simulink model "CDMA2000sint_C_etapa4"  (R2012b)
settings: Solver=ode45  StartTime=0.0  StopTime=200  RelTol=1e-3
libraries: commcnvintrlv2 x2, commcnvcod2 x2, commrandsrc2 x1, commsink2 x1
settings Model: Creator=Oti  LastModifiedBy=student
settings DataIOCC: SignalLoggingSaveFormat=ModelDataLogs
settings DebuggingCC: FcnCallInpInsideContextMsg=UseLocalSettings
settings GRTTargetCC: CombineOutputUpdateFcns=off  GRTInterface=on

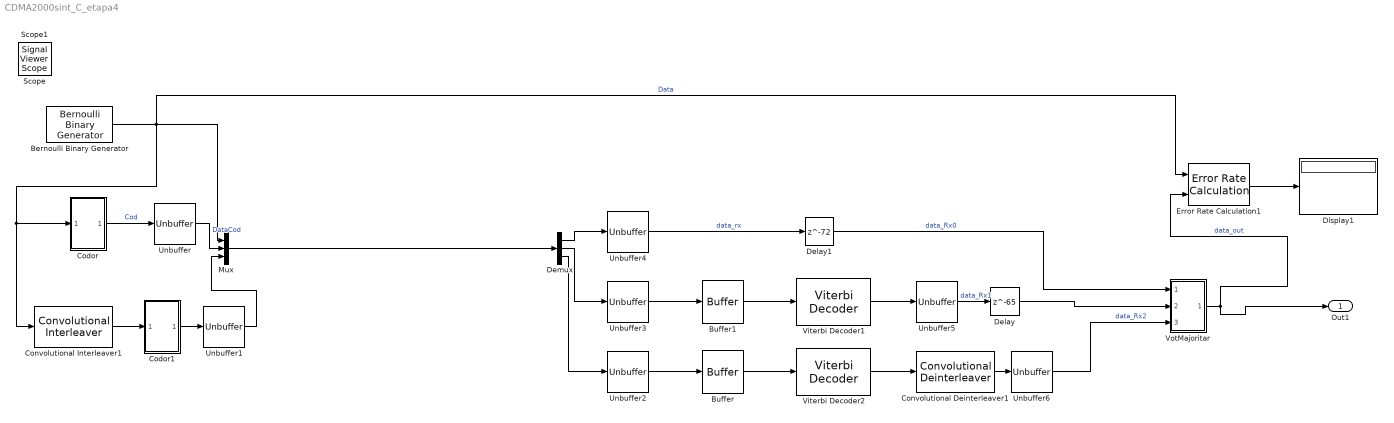
== system CDMA2000sint_C_etapa4 ==
  Bernoulli Binary Generator : commrandsrc2/Bernoulli Binary Generator  P=0.5  seed=61  Ts=1  frameBased=off  sampPerFrame=1  orient=off  outDataType=boolean
  Buffer : Buffer  N=3  TreatMby1Signals=One channel
  Buffer1 : Buffer  N=3  TreatMby1Signals=One channel
  Codor : Subsystem
  Codor1 : Subsystem
  Convolutional Deinterleaver1 : commcnvintrlv2/Convolutional Deinterleaver  N=6  B=2  ic=0
  Convolutional Interleaver1 : commcnvintrlv2/Convolutional Interleaver  N=6  B=2  ic=0
  Delay : Delay  DelayLength=65  SampleTime=1
  Delay1 : Delay  DelayLength=72  SampleTime=1
  Demux : Demux  Outputs=3
  Display1 : Display
  Error Rate Calculation1 : commsink2/Error Rate Calculation  N=72  st_delay=0  cp_mode=Entire frame  subframe=[]  PMode=Port  WsName=ErrorVec  RsMode2=off  stop=off  numErr=100  maxBits=1e6
  Mux : Mux  Inputs=3
  Unbuffer{,1..6} (7 alike) : Unbuffer  SampleBasedProcessing=Same as frame based
  Viterbi Decoder1 : commcnvcod2/Viterbi Decoder  trellis=poly2trellis(4, [13 15 17], 13)  isPunctured=off  punctureVector=[1; 1; 0; 1; 0; 1]  erasures=off  dectype=Hard decision  runSigValErrCheck=off  nsdecb=4  smWordLength=16  tbdepth=6  opmode=Continuous  reset=off  outDataType=boolean  delayedResetAction=off
  Viterbi Decoder2 : commcnvcod2/Viterbi Decoder  trellis=poly2trellis(4, [13 15 17], 13)  isPunctured=off  punctureVector=[1; 1; 0; 1; 0; 1]  erasures=off  dectype=Hard decision  runSigValErrCheck=off  nsdecb=4  smWordLength=16  tbdepth=11  opmode=Continuous  reset=off  outDataType=boolean  delayedResetAction=off
  "VotMajoritar " : Subsystem
  Out1 : Outport
  Scope : SignalViewerScope  IOType=viewer  NumInputPorts=2  RefreshTime=0.035000
      settings: ShowDataMarkers=on  YMin=-5~-5  YMax=5~5
  Scope1 : SignalViewerScope  IOType=viewer  NumInputPorts=4  ZoomMode=xonly  LegendLocations=|  RefreshTime=0.035000
      | 0.89307     0.91669    0.091016    0.035112
      | 0.90792     0.67618    0.076172    0.035112
      | 0.89307     0.43708    0.091016    0.035112
      |  0.8962     0.19658    0.087891    0.035112
      settings: TickLabels=on  ShowLegends=on  YMin=-5~-5~-5~-5  YMax=5~5~5~5
  wires:
  Bernoulli Binary Generator/1 -> Codor/1(In1), Convolutional Interleaver1/1, Mux/1, Error Rate Calculation1/1  "Data"
  Codor/1(Out2) -> Unbuffer/1  "Cod"
  Codor1/1(Out2) -> Unbuffer1/1
  Convolutional Interleaver1/1 -> Codor1/1(In1)
  Unbuffer1/1 -> Mux/3
  Demux/1 -> Unbuffer4/1
  Demux/2 -> Unbuffer3/1
  Demux/3 -> Unbuffer2/1
  Unbuffer3/1 -> Buffer1/1
  Unbuffer2/1 -> Buffer/1
  Buffer1/1 -> Viterbi Decoder1/1
  Buffer/1 -> Viterbi Decoder2/1
  Viterbi Decoder2/1 -> Convolutional Deinterleaver1/1
  Viterbi Decoder1/1 -> Unbuffer5/1
  Convolutional Deinterleaver1/1 -> Unbuffer6/1
  Unbuffer4/1 -> Delay1/1  "data_rx"
  Delay1/1 -> "VotMajoritar "/1(In1)  "data_Rx0"
  Unbuffer5/1 -> Delay/1  "data_Rx1"
  "VotMajoritar "/1(Out1) -> Out1/1, Error Rate Calculation1/2  "data_out"
  Unbuffer6/1 -> "VotMajoritar "/3(In3)  "data_Rx2"
  Error Rate Calculation1/1 -> Display1/1
  Unbuffer/1 -> Mux/2  "DataCod"
  Delay/1 -> "VotMajoritar "/2(In2)
  Mux/1 -> Demux/1

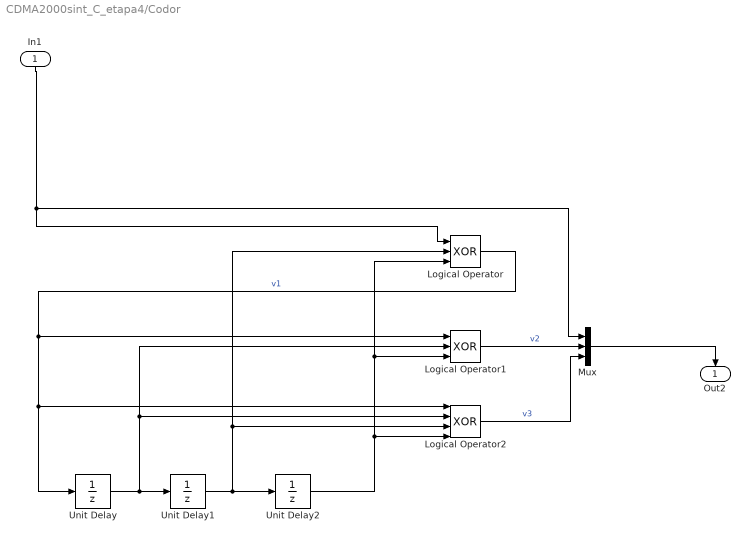
== system CDMA2000sint_C_etapa4/Codor ==
  In1 : Inport
  Logical Operator : Logic  Operator=XOR  Inputs=3  IconShape=distinctive  AllPortsSameDT=off  OutDataTypeStr=boolean
  Logical Operator1 : Logic  Operator=XOR  Inputs=3  IconShape=distinctive  AllPortsSameDT=off  OutDataTypeStr=boolean
  Logical Operator2 : Logic  Operator=XOR  Inputs=4  IconShape=distinctive  AllPortsSameDT=off  OutDataTypeStr=boolean
  Mux : Mux  Inputs=3
  Unit Delay : UnitDelay  SampleTime=-1
  Unit Delay1 : UnitDelay  SampleTime=-1
  Unit Delay2 : UnitDelay  SampleTime=-1
  Out2 : Outport
  wires:
  Logical Operator2/1 -> Mux/3  "v3"
  Logical Operator/1 -> Logical Operator1/1, Logical Operator2/1, Unit Delay/1  "v1"
  Unit Delay/1 -> Logical Operator1/2, Logical Operator2/2, Unit Delay1/1
  Unit Delay1/1 -> Logical Operator/2, Logical Operator2/3, Unit Delay2/1
  Mux/1 -> Out2/1
  In1/1 -> Mux/1, Logical Operator/1
  Logical Operator1/1 -> Mux/2  "v2"
  Unit Delay2/1 -> Logical Operator1/3, Logical Operator/3, Logical Operator2/4

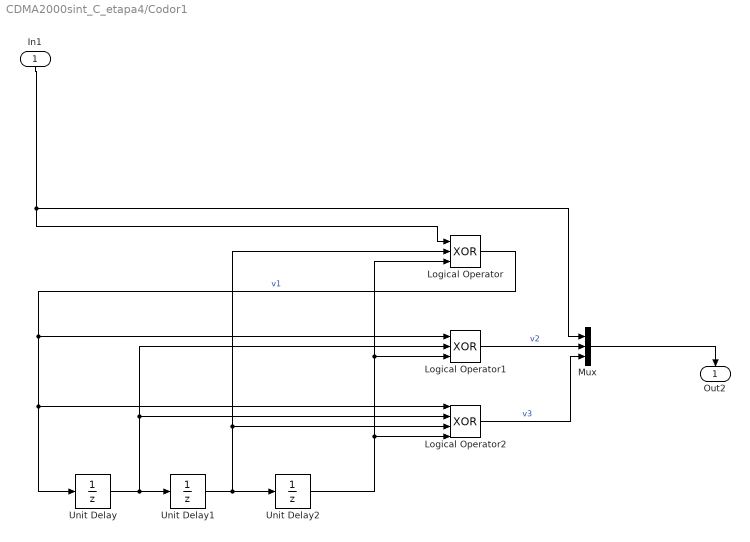
== system CDMA2000sint_C_etapa4/Codor1 ==
  In1 : Inport
  Logical Operator : Logic  Operator=XOR  Inputs=3  IconShape=distinctive  AllPortsSameDT=off  OutDataTypeStr=boolean
  Logical Operator1 : Logic  Operator=XOR  Inputs=3  IconShape=distinctive  AllPortsSameDT=off  OutDataTypeStr=boolean
  Logical Operator2 : Logic  Operator=XOR  Inputs=4  IconShape=distinctive  AllPortsSameDT=off  OutDataTypeStr=boolean
  Mux : Mux  Inputs=3
  Unit Delay : UnitDelay  SampleTime=-1
  Unit Delay1 : UnitDelay  SampleTime=-1
  Unit Delay2 : UnitDelay  SampleTime=-1
  Out2 : Outport
  wires:
  Logical Operator2/1 -> Mux/3  "v3"
  Logical Operator/1 -> Logical Operator1/1, Logical Operator2/1, Unit Delay/1  "v1"
  Unit Delay/1 -> Logical Operator1/2, Logical Operator2/2, Unit Delay1/1
  Unit Delay1/1 -> Logical Operator/2, Logical Operator2/3, Unit Delay2/1
  Mux/1 -> Out2/1
  In1/1 -> Mux/1, Logical Operator/1
  Logical Operator1/1 -> Mux/2  "v2"
  Unit Delay2/1 -> Logical Operator1/3, Logical Operator/3, Logical Operator2/4

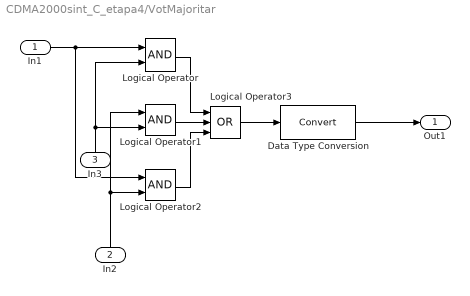
== system CDMA2000sint_C_etapa4/VotMajoritar  ==
  In1 : Inport
  In2 : Inport  Port=2
  In3 : Inport  Port=3
  Data Type Conversion : DataTypeConversion
  Logical Operator : Logic  AllPortsSameDT=off  OutDataTypeStr=boolean
  Logical Operator1 : Logic  AllPortsSameDT=off  OutDataTypeStr=boolean
  Logical Operator2 : Logic  AllPortsSameDT=off  OutDataTypeStr=boolean
  Logical Operator3 : Logic  Operator=OR  Inputs=3  AllPortsSameDT=off  OutDataTypeStr=boolean
  Out1 : Outport
  wires:
  Logical Operator1/1 -> Logical Operator3/2
  Logical Operator3/1 -> Data Type Conversion/1
  In3/1 -> Logical Operator1/2, Logical Operator/2
  In1/1 -> Logical Operator2/1, Logical Operator/1
  Logical Operator2/1 -> Logical Operator3/3
  In2/1 -> Logical Operator2/2, Logical Operator1/1
  Data Type Conversion/1 -> Out1/1
  Logical Operator/1 -> Logical Operator3/1
